simulink model "Act_1"  (R2017b)
settings: Solver=ode2  StartTime=0.0  StopTime=20  FixedStep=0.001  RelTol=1e-3
settings Model: Creator=Marco  LastModifiedBy=Marco

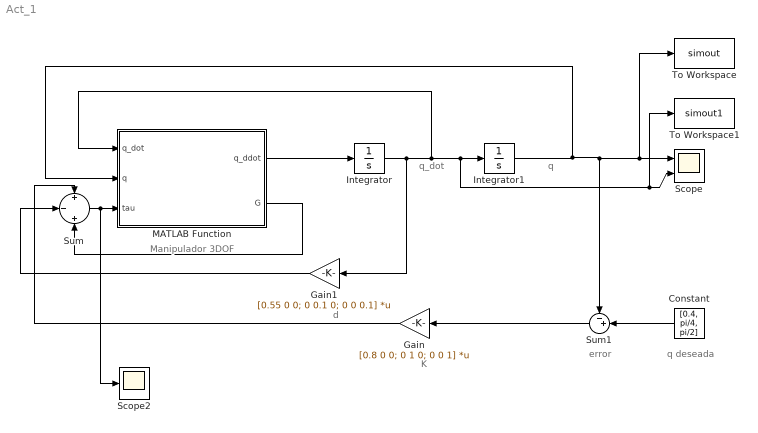
== system Act_1 ==
  note: error
  note: Manipulador 3DOF
  note: d
  note: K
  note: q deseada
  note: q
  note: q_dot
  Constant : Constant  Value=[0.4, pi/4, pi/2]
  Gain : Gain  Gain=[0.8 0 0; 0 1 0; 0 0 1]  Multiplication=Matrix(K*u)
  Gain1 : Gain  Gain=[0.55 0 0; 0 0.1 0; 0 0 0.1]  Multiplication=Matrix(K*u)
  Integrator : Integrator  InitialCondition=[0; 0; 0]
  Integrator1 : Integrator  InitialCondition=[0.2; 0; 0]
  MATLAB Function : MATLAB Function  TreatAsAtomicUnit=on
  Scope : Scope  NumInputPorts=2
  Scope2 : Scope
  Sum : Sum  Inputs=+|-|+
  Sum1 : Sum  Inputs=-+|
  To Workspace : ToWorkspace  VariableName=simout  SaveFormat=Timeseries  SampleTime=-1
  To Workspace1 : ToWorkspace  VariableName=simout1  SaveFormat=Timeseries  SampleTime=-1
  wires:
  MATLAB Function/1(q_ddot) -> Integrator/1
  Integrator/1 -> Gain1/1, MATLAB Function/1(q_dot), To Workspace1/1, Scope/2, Integrator1/1
  Integrator1/1 -> Sum1/1, To Workspace/1, Scope/1, MATLAB Function/2(q)
  Sum/1 -> Scope2/1, MATLAB Function/3(tau)
  Constant/1 -> Sum1/2
  Sum1/1 -> Gain/1
  Gain/1 -> Sum/1
  Gain1/1 -> Sum/2
  MATLAB Function/2(G) -> Sum/3

== matlab function Act_1/MATLAB Function ==
  data: q_dot input; q input; q_ddot output; tau input; G output
function [q_ddot, G]= manipulador(q_dot,q,tau)
%Valores del robot
g = 9.81; %m/s^2
l2 = 0.3; %m
lc2 = 0.15; %m
lc3 = 0.15; %m
m1 = 0.2; %Kg
m2 = 0.2; %Kg
m3 = 0.2; %Kg
I2 = 0.001; %Kg*m^2
I3 = 0.001; %Kg*m^2

%---------------------------Matriz de Inercias----------------------------%
m11 = m1/4 + m2 + m3;
m12 = lc2*m2*cos(q(2)) + m3*cos(q(2))*(l2 + lc3*cos(q(3)));
m13 = lc3*m3*sin(q(2))*sin(q(3));
m21 = lc2*m2*cos(q(2)) + m3*cos(q(2))*(l2 + lc3*cos(q(3)));
m22 = I2 + I3 + (l2^2)*m3 + (lc2^2)*m2 + (lc3^2)*m3*cos(q(3))^2 + 2*l2*lc3*m3*cos(q(3));
m23 = 0;
m31 = -lc3*m3*sin(q(2))*sin(q(3));
m32 = 0; 
m33 = m3*(lc3^2) + I3;

M = [m11 m12 m13;
     m21 m22 m23;
     m31 m32 m33];
%----------------------------Matriz de Coriolis---------------------------%

c11 = 0;
c12 = - q_dot(2)*(lc2*m2*sin(q(2)) + m3*sin(q(2))*(l2 + lc3*cos(q(3)))) - lc3*m3*q_dot(3)*cos(q(2))*sin(q(3));
c13 = -lc3*m3*(q_dot(2)*cos(q(2))*sin(q(3)) + q_dot(3)*cos(q(3))*sin(q(2)));
c21 = 0;
c22 = -(lc3*m3*q_dot(3)*(lc3*sin(2*q(3)) + 2*l2*sin(q(3))))/2;
c23 = -(lc3*m3*q_dot(2)*(lc3*sin(2*q(3)) + 2*l2*sin(q(3))))/2;
c31 = 0;
c32 = (lc3*m3*q_dot(1)*(lc3*sin(2*q(3)) + 2*l2*sin(q(3))))/2;
c33 = 0;

C = [c11 c12 c13;
     c21 c22 c23;
     c31 c32 c33];
%----------------------------Vector de Gravedad---------------------------%
g11 = g*((m1/2)+m2+m3);
g21 = g*(lc3*m3*cos(q(3))+l2*m3+lc2*m2)*cos(q(2));
g31 = -g*lc3*m3*sin(q(2))*sin(q(3));

G = [g11;
     g21;
     g31];
 
q_ddot = M\(tau-C*q_dot-G);
